simulink model "Task_3"  (R2022b)
settings: Solver=VariableStepAuto  StartTime=0.0  StopTime=10.0  RelTol=1e-3
settings Model: Creator=Abanob_Sameh  LastModifiedBy=Abanob_Sameh

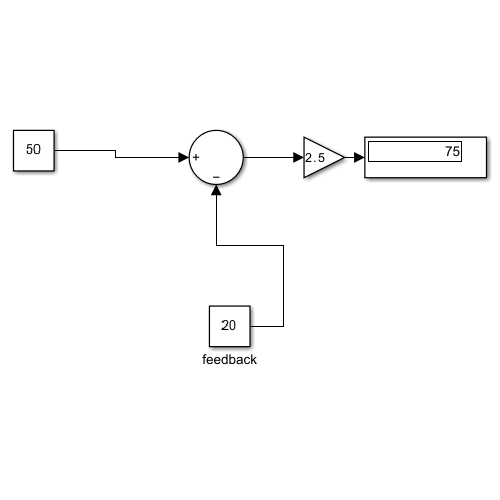
[thumbnail: Simulink's stored preview of the top-level diagram]
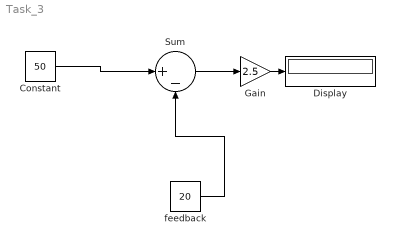
== system Task_3 ==
  Constant : Constant  Value=50
  Display : Display
  Gain : Gain  Gain=2.5
  Sum : Sum  Inputs=|+-
  feedback : Constant  Value=20
  wires:
  Constant/1 -> Sum/1
  Sum/1 -> Gain/1
  Gain/1 -> Display/1
  feedback/1 -> Sum/2
